simulink model "CM4_ADC_All_v2"  (R2020b)
settings: Solver=FixedStepDiscrete  StartTime=0.0  StopTime=inf  FixedStep=0.05  RelTol=1e-3  EnableMultiTasking=on
libraries: simulink x3, embdlinuxlib x1, raspberrypiCommlib x1
settings Model: ModifiedByFormat=The MathWorks Inc.  SimulationMode=external  EnablePacing=on  Creator=The MathWorks, Inc.  LastModifiedBy=The MathWorks Inc.
settings SolverCC: PositivePriorityOrder=on
settings DataIOCC: LimitDataPoints=on  SaveFormat=Array  ReturnWorkspaceOutputs=off
settings OptimizationCC: LifeSpan=1  MaxStackSize=64
settings DebuggingCC: UnderspecifiedInitializationDetection=Classic  MergeDetectMultiDrivingBlocksExec=none  SolverPrmCheckMsg=warning  AllowSymbolicDim=off  SFUnexpectedBacktrackingDiag=warning  SFNoUnconditionalDefaultTransitionDiag=warning  SFExecutionAtInitializationDiag=none  ArithmeticOperatorsInVariantConditions=warning
settings HardwareCC: ProdBitPerPointer=32  ProdBitPerSizeT=32  ProdBitPerPtrDiffT=32  ProdLargestAtomicInteger=Long  ProdLargestAtomicFloat=Double  ProdWordSize=32  ProdLongLongMode=on  ProdHWDeviceType=ARM Compatible->ARM Cortex
settings SFSimCC: SimUseLocalCustomCode=off  MATLABDynamicMemAlloc=off  CustomCodeUndefinedFunction=UseInterfaceOnly
settings RTWCC: Description=Embedded Coder  SystemTargetFile=ert.tlc  HardwareBoard=Raspberry Pi  TemplateMakefile=ert_default_tmf  RTWUseLocalCustomCode=off  Toolchain=GNU GCC Raspberry Pi
settings CodeAppCC: StateflowObjectComments=on
settings ERTTargetCC: MultiwordLength=2048  ERTCustomFileBanners=off  MatFileLogging=on  SupportContinuousTime=on  SupportNonInlinedSFcns=on  RemoveResetFunc=off  ModelStepFunctionPrototypeControlCompliant=off  ConvertIfToSwitch=off  SuppressUnreachableDefaultCases=off
settings ConfigComp: CovMetricSettings=dw  CovSaveCumulativeToWorkspaceVar=on  CovSaveSingleToWorkspaceVar=on  CovExternalEMLEnable=off  CovSFcnEnable=off

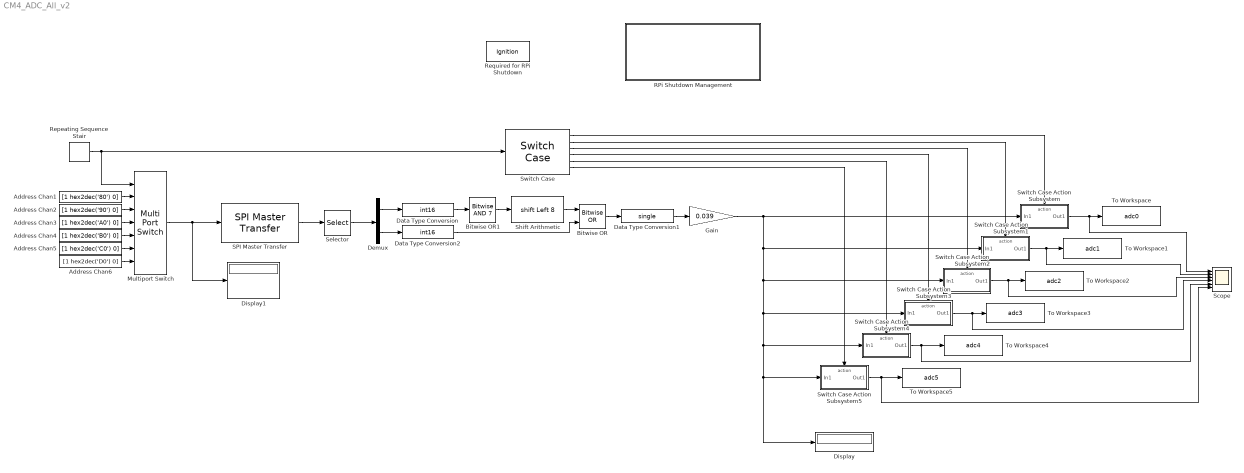
== system CM4_ADC_All_v2 ==
  Address Chan1 : Constant  Value=[1 hex2dec('80') 0]  OutDataTypeStr=uint8
  Address Chan2 : Constant  Value=[1 hex2dec('90') 0]  OutDataTypeStr=uint8
  Address Chan3 : Constant  Value=[1 hex2dec('A0') 0]  OutDataTypeStr=uint8
  Address Chan4 : Constant  Value=[1 hex2dec('B0') 0]  OutDataTypeStr=uint8
  Address Chan5 : Constant  Value=[1 hex2dec('C0') 0]  OutDataTypeStr=uint8
  Address Chan6 : Constant  Value=[1 hex2dec('D0') 0]  OutDataTypeStr=uint8
  Bitwise OR : simulink/Logic and Bit Operations/Bitwise Operator  logicop=OR  UseBitMask=off  NumInputPorts=2  BitMask=bin2dec('11011001')  BitMaskRealWorld=Stored Integer
  Bitwise OR1 : simulink/Logic and Bit Operations/Bitwise Operator  logicop=AND  UseBitMask=on  BitMask=7  BitMaskRealWorld=Stored Integer
  Data Type Conversion : DataTypeConversion  OutDataTypeStr=int16
  Data Type Conversion1 : DataTypeConversion  OutDataTypeStr=single
  Data Type Conversion2 : DataTypeConversion  OutDataTypeStr=int16
  Demux : Demux  Outputs=2
  Display : Display
  Display1 : Display
  Gain : Gain  Gain=0.039
  Multiport Switch : MultiPortSwitch  DataPortOrder=Zero-based contiguous  Inputs=6  zeroidx=on  OutDataTypeStr=uint8
  RPi Shutdown Management : Subsystem
  Repeating Sequence Stair : simulink/Sources/Repeating Sequence Stair  OutValues=[0 1 2 3 4 5]'  tsamp=-1  OutMin=[]  OutMax=[]  OutDataTypeStr=double  OutputDataTypeScalingMode=double  OutDataType=fixdt(0,8)  ConRadixGroup=Best Precision: Vector-wise  OutScaling=2^-12
  Required for RPi Shutdown : DataStoreMemory  DataStoreName=Ignition  ReadBeforeWriteMsg=warning  WriteAfterWriteMsg=warning  WriteAfterReadMsg=warning  ShowAdditionalParam=off  OutDataTypeStr=uint8
  SPI Master Transfer : raspberrypiCommlib/SPI Master Transfer  BoardProperty=Pi 4 Model B  SSPin=SPI0_CE1  SPIModule=uint32(0)  Mode=Master  BusSpeed=1000000  Pin=uint32(0)  FirstBitToTransfer=Most significant bit (MSB)  ClockMode=0  BlockFunction=Transfer  RegisterAddress=0  OutputDataType=int8  OutputDataLength=1
      settings: SourceProductBaseCode=RASPPI
  Scope : Scope  NumInputPorts=6
  Selector : Selector  InputPortWidth=3  IndexOptions=Index vector (dialog)  Indices=[2 3]  OutputSizes=1
  Shift Arithmetic : ArithShift  BitShiftNumber=8  BitShiftDirection=Left
  Switch Case : SwitchCase  CaseConditions={0,1,2,3,4,5}  ShowDefaultCase=off
  Switch Case Action Subsystem : Subsystem  TreatAsAtomicUnit=on
  Switch Case Action Subsystem1 : Subsystem  TreatAsAtomicUnit=on
  Switch Case Action Subsystem2 : Subsystem  TreatAsAtomicUnit=on
  Switch Case Action Subsystem3 : Subsystem  TreatAsAtomicUnit=on
  Switch Case Action Subsystem4 : Subsystem  TreatAsAtomicUnit=on
  Switch Case Action Subsystem5 : Subsystem  TreatAsAtomicUnit=on
  To Workspace : ToWorkspace  VariableName=adc0  SampleTime=-1
      settings: Save2DSignal=2-D array (concatenate along first dimension)
  To Workspace1 : ToWorkspace  VariableName=adc1  SampleTime=-1
      settings: Save2DSignal=2-D array (concatenate along first dimension)
  To Workspace2 : ToWorkspace  VariableName=adc2  SampleTime=-1
      settings: Save2DSignal=2-D array (concatenate along first dimension)
  To Workspace3 : ToWorkspace  VariableName=adc3  SampleTime=-1
      settings: Save2DSignal=2-D array (concatenate along first dimension)
  To Workspace4 : ToWorkspace  VariableName=adc4  SampleTime=-1
      settings: Save2DSignal=2-D array (concatenate along first dimension)
  To Workspace5 : ToWorkspace  VariableName=adc5  SampleTime=-1
      settings: Save2DSignal=2-D array (concatenate along first dimension)
  wires:
  Address Chan2/1 -> Multiport Switch/3
  Switch Case/3 -> Switch Case Action Subsystem2/Action
  Address Chan6/1 -> Multiport Switch/7
  Switch Case/6 -> Switch Case Action Subsystem5/Action
  Selector/1 -> Demux/1
  Switch Case Action Subsystem5/1(Out1) -> Scope/6, To Workspace5/1
  Data Type Conversion2/1 -> Bitwise OR/2
  Switch Case Action Subsystem/1(Out1) -> Scope/1, To Workspace/1
  Switch Case/5 -> Switch Case Action Subsystem4/Action
  Gain/1 -> Display/1, Switch Case Action Subsystem5/1(In1), Switch Case Action Subsystem4/1(In1), Switch Case Action Subsystem3/1(In1), Switch Case Action Subsystem2/1(In1), Switch Case Action Subsystem1/1(In1), Switch Case Action Subsystem/1(In1)
  Multiport Switch/1 -> SPI Master Transfer/1, Display1/1
  Switch Case/4 -> Switch Case Action Subsystem3/Action
  Switch Case Action Subsystem4/1(Out1) -> Scope/5, To Workspace4/1
  Switch Case Action Subsystem2/1(Out1) -> Scope/3, To Workspace2/1
  Data Type Conversion/1 -> Bitwise OR1/1
  Bitwise OR1/1 -> Shift Arithmetic/1
  Switch Case/2 -> Switch Case Action Subsystem1/Action
  Demux/2 -> Data Type Conversion2/1
  Switch Case/1 -> Switch Case Action Subsystem/Action
  Switch Case Action Subsystem1/1(Out1) -> Scope/2, To Workspace1/1
  Address Chan3/1 -> Multiport Switch/4
  Address Chan4/1 -> Multiport Switch/5
  Data Type Conversion1/1 -> Gain/1
  Shift Arithmetic/1 -> Bitwise OR/1
  Demux/1 -> Data Type Conversion/1
  Address Chan5/1 -> Multiport Switch/6
  Repeating Sequence Stair/1 -> Multiport Switch/1, Switch Case/1
  Address Chan1/1 -> Multiport Switch/2
  Switch Case Action Subsystem3/1(Out1) -> Scope/4, To Workspace3/1
  SPI Master Transfer/1 -> Selector/1
  Bitwise OR/1 -> Data Type Conversion1/1

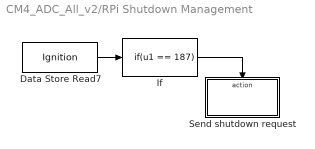
== system CM4_ADC_All_v2/RPi Shutdown Management ==
  Data Store Read7 : DataStoreRead  DataStoreName=Ignition
  If : If  IfExpression=u1 == 187  ShowElse=off
  Send shutdown request : Subsystem  TreatAsAtomicUnit=on
  wires:
  If/1 -> Send shutdown request/Action
  Data Store Read7/1 -> If/1

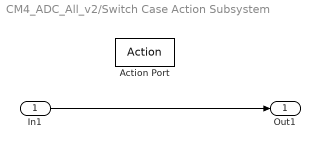
== system CM4_ADC_All_v2/Switch Case Action Subsystem ==
  In1 : Inport
  Action Port : ActionPort  ActionPortLabel=case [ 0 ]:
  Out1 : Outport
  wires:
  In1/1 -> Out1/1

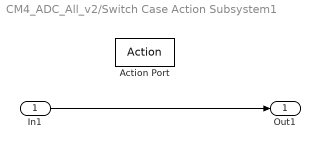
== system CM4_ADC_All_v2/Switch Case Action Subsystem1 ==
  In1 : Inport
  Action Port : ActionPort  ActionPortLabel=case [ 1 ]:
  Out1 : Outport
  wires:
  In1/1 -> Out1/1

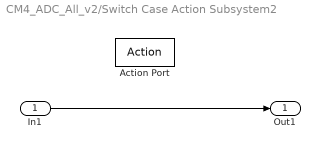
== system CM4_ADC_All_v2/Switch Case Action Subsystem2 ==
  In1 : Inport
  Action Port : ActionPort  ActionPortLabel=case [ 2 ]:
  Out1 : Outport
  wires:
  In1/1 -> Out1/1

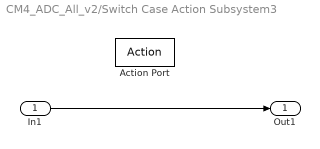
== system CM4_ADC_All_v2/Switch Case Action Subsystem3 ==
  In1 : Inport
  Action Port : ActionPort  ActionPortLabel=case [ 3 ]:
  Out1 : Outport
  wires:
  In1/1 -> Out1/1

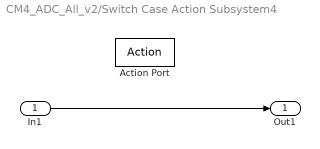
== system CM4_ADC_All_v2/Switch Case Action Subsystem4 ==
  In1 : Inport
  Action Port : ActionPort  ActionPortLabel=case [ 4 ]:
  Out1 : Outport
  wires:
  In1/1 -> Out1/1

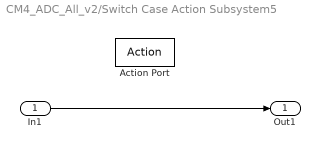
== system CM4_ADC_All_v2/Switch Case Action Subsystem5 ==
  In1 : Inport
  Action Port : ActionPort  ActionPortLabel=case [ 5 ]:
  Out1 : Outport
  wires:
  In1/1 -> Out1/1

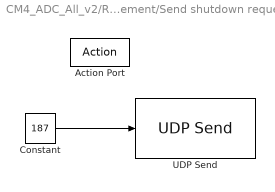
== system CM4_ADC_All_v2/RPi Shutdown Management/Send shutdown request ==
  Action Port : ActionPort  ActionPortLabel=if(u1 == 187)
  Constant : Constant  Value=187  OutDataTypeStr=uint8
  UDP Send : embdlinuxlib/UDP Send  remoteURL='127.0.0.1'  remotePort=5005  localURL='255.255.255.255'  localPortSource=Automatically determine  localPort=-1  sampletime=-1  blockPlatform=Raspberry Pi  separateLengthPort=0
      settings: SourceProductBaseCode=SC_BEAGLEBONE_BLUE,NVIDIA,RASPPI
  wires:
  Constant/1 -> UDP Send/1
